simulink model "parallel_lht_accumulator"  (R2019b)
settings: Solver=FixedStepDiscrete  StartTime=0.0  StopTime=inf  RelTol=1e-3
InitFcn:
  | parallel_lht_setup;
StopFcn:
  | parallel_lht_accumulator_compare;
undefined symbols (not defined in the file or in its folder): bt, height, nTheta, width
libraries: hdlsllib x21, simulink x18, dspsrcs4 x1
(part 1 of 2)
settings Model: DataTypeOverride=Off  SimulationMode=rapid-accelerator  Creator=rgb11127  LastModifiedBy=rgb11127
settings DataIOCC: SaveOutput=off  SaveTime=off
settings OptimizationCC: BlockReduction=off  ConditionallyExecuteInputs=off  DefaultParameterBehavior=Inlined
settings DebuggingCC: AlgebraicLoopMsg=error  SingleTaskRateTransMsg=error
settings HardwareCC: ProdBitPerPointer=32  ProdBitPerSizeT=32  ProdBitPerPtrDiffT=32  ProdLargestAtomicFloat=None  ProdIntDivRoundTo=Undefined  ProdEndianess=Unspecified  ProdWordSize=32  ProdHWDeviceType=ASIC/FPGA->ASIC/FPGA  TargetBitPerPointer=64  TargetBitPerSizeT=64  TargetBitPerPtrDiffT=64  TargetLongLongMode=on  TargetIntDivRoundTo=Zero  TargetEndianess=LittleEndian  TargetWordSize=64  TargetHWDeviceType=Custom Processor->MATLAB Host Computer  ProdEqTarget=off

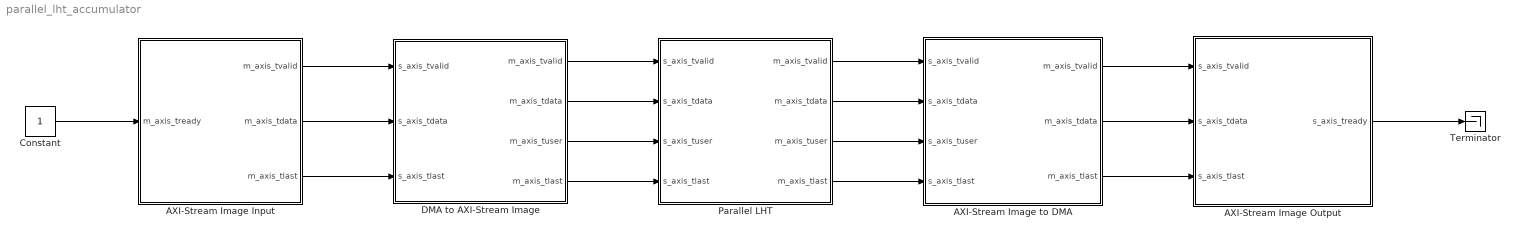
== system parallel_lht_accumulator ==
  AXI-Stream Image Input : Subsystem  mask{image=bt.inputImage, clk=1/150e6}
      mask prompts: image "Input Image:"; clk "Clock Rate:"
      mask init:
      | [height, width] = size(image);
      mask DialogControl DescGroupVar Prompt: AXI-Stream Image Input
      mask DialogControl DescTextVar Prompt: This block simulates an AXI-Stream image input for interfacing to a hardware accelerator or IP Core.
      mask DialogControl ParameterGroupVar Prompt: Main
  AXI-Stream Image Output : Subsystem  mask{height=bt.nRho, width=bt.nTheta, clk=1/150e6, d=0}
      mask prompts: height "Image Height:"; width "Image Width:"; clk "Clock Rate:"; d "Frame Capture Number"
      mask DialogControl DescGroupVar Prompt: AXI-Stream Image Output
      mask DialogControl DescTextVar Prompt: Image output using the AXI-Stream interface. Simulates an AXI DMA write channel.
      mask DialogControl ParameterGroupVar Prompt: Main
  AXI-Stream Image to DMA : Subsystem  mask{height=bt.nRho, width=bt.nTheta}
      mask prompts: height "Image Height"; width "Image Width"
      mask DialogControl DescGroupVar Prompt: AXI-Stream Image to DMA
      mask DialogControl DescTextVar Prompt: Converts from the AXI-Stream video standard to AXI-Stream DMA packet.
      mask DialogControl Container2 Prompt: Main
  Constant : Constant  OutDataTypeStr=boolean  SampleTime=-1
  DMA to AXI-Stream Image : Subsystem  mask{height=bt.height, width=bt.width, b=1}
      mask prompts: height "Image Height:"; width "Image Width:"; b "Bits"
      mask DialogControl DescGroupVar Prompt: DMA to AXI-Stream Image
      mask DialogControl DescTextVar Prompt: Converts an DMA AXI-Stream packet to the AXI-Stream video standard.
      mask DialogControl Container2 Prompt: Main
  Parallel LHT : Subsystem
  Terminator : Terminator
  wires:
  Constant/1 -> AXI-Stream Image Input/1(m_axis_tready)
  AXI-Stream Image Input/1(m_axis_tvalid) -> DMA to AXI-Stream Image/1(s_axis_tvalid)
  AXI-Stream Image Input/2(m_axis_tdata) -> DMA to AXI-Stream Image/2(s_axis_tdata)
  AXI-Stream Image Input/3(m_axis_tlast) -> DMA to AXI-Stream Image/3(s_axis_tlast)
  AXI-Stream Image to DMA/1(m_axis_tvalid) -> AXI-Stream Image Output/1(s_axis_tvalid)
  AXI-Stream Image to DMA/2(m_axis_tdata) -> AXI-Stream Image Output/2(s_axis_tdata)
  AXI-Stream Image to DMA/3(m_axis_tlast) -> AXI-Stream Image Output/3(s_axis_tlast)
  AXI-Stream Image Output/1(s_axis_tready) -> Terminator/1
  DMA to AXI-Stream Image/1(m_axis_tvalid) -> Parallel LHT/1(s_axis_tvalid)
  DMA to AXI-Stream Image/2(m_axis_tdata) -> Parallel LHT/2(s_axis_tdata)
  DMA to AXI-Stream Image/3(m_axis_tuser) -> Parallel LHT/3(s_axis_tuser)
  DMA to AXI-Stream Image/4(m_axis_tlast) -> Parallel LHT/4(s_axis_tlast)
  Parallel LHT/1(m_axis_tvalid) -> AXI-Stream Image to DMA/1(s_axis_tvalid)
  Parallel LHT/2(m_axis_tdata) -> AXI-Stream Image to DMA/2(s_axis_tdata)
  Parallel LHT/3(m_axis_tuser) -> AXI-Stream Image to DMA/3(s_axis_tuser)
  Parallel LHT/4(m_axis_tlast) -> AXI-Stream Image to DMA/4(s_axis_tlast)

== system parallel_lht_accumulator/AXI-Stream Image Input ==
  m_axis_tready : Inport
  Compare To Constant : simulink/Logic and Bit Operations/Compare To Constant  relop===  const=height*width-1  OutDataTypeStr=boolean
  Data Type Conversion : DataTypeConversion  OutDataTypeStr=uint32
  HDL Counter : hdlsllib/Sources/HDL Counter  CountType=Count limited  CountInit=0  CountStep=1  CountMax=width*height-1  CountFromType=Initial value  CountFrom=0  CountResetPort=off  CountLoadPort=off  CountEnbPort=on  CountDirPort=off  CountDataType=Unsigned  CountWordLen=ceil(log2(width*height))  CountFracLen=0  CountSampTime=1
      settings: SourceProductName=Simulink
  Master AXI-Stream FIFO : Subsystem  mask{depth=32}
      mask prompts: depth "FIFO Depth:"
      mask DialogControl DescGroupVar Prompt: Master AXI-Stream FIFO
      mask DialogControl DescTextVar Prompt: A custom AXI-Stream FIFO for interfacing to write channel AXI DMAs.
      mask DialogControl ParameterGroupVar Prompt: Main
  Synchronous Image Source : Subsystem
  m_axis_tvalid : Outport
  m_axis_tdata : Outport  Port=2
  m_axis_tlast : Outport  Port=3
  wires:
  Master AXI-Stream FIFO/2(m_axis_tdata) -> m_axis_tdata/1
  Master AXI-Stream FIFO/3(m_axis_tlast) -> m_axis_tlast/1
  m_axis_tready/1 -> Master AXI-Stream FIFO/4(m_axis_tready)
  Master AXI-Stream FIFO/4(s_axis_tready) -> HDL Counter/1, Master AXI-Stream FIFO/1(s_axis_tvalid), Synchronous Image Source/Enable
  Compare To Constant/1 -> Master AXI-Stream FIFO/3(s_axis_tlast)
  Data Type Conversion/1 -> Master AXI-Stream FIFO/2(s_axis_tdata)
  Master AXI-Stream FIFO/1(m_axis_tvalid) -> m_axis_tvalid/1
  Synchronous Image Source/1(Pixel) -> Data Type Conversion/1
  HDL Counter/1 -> Compare To Constant/1

== system parallel_lht_accumulator/AXI-Stream Image Output ==
  s_axis_tvalid : Inport
  s_axis_tdata : Inport  Port=2
  s_axis_tlast : Inport  Port=3
  AND1 : Logic  IconShape=distinctive  AllPortsSameDT=off  OutDataTypeStr=boolean
  Compare To Constant4 : simulink/Logic and Bit Operations/Compare To Constant  relop===  const=(height)*width-1  OutDataTypeStr=boolean
  Constant : Constant  OutDataTypeStr=boolean  SampleTime=-1
  Delay2 : Delay  DelayLength=d  ShowEnablePort=on
      settings: InputPortMap=u0,e6
  Pixel to Workspace : Subsystem
  Stop Simulation1 : Stop
  Terminator : Terminator
  Total Samples Counter : hdlsllib/Sources/HDL Counter  CountType=Count limited  CountInit=0  CountStep=1  CountMax=(height)*width-1  CountFromType=Initial value  CountFrom=0  CountResetPort=off  CountLoadPort=off  CountEnbPort=on  CountDirPort=off  CountDataType=Unsigned  CountWordLen=ceil(log2((height)*width+1))  CountFracLen=0  CountSampTime=1
      settings: SourceProductName=Simulink
  s_axis_tready : Outport  VectorParamsAs1DForOutWhenUnconnected=off
  wires:
  s_axis_tdata/1 -> Pixel to Workspace/1(Pixel In)
  s_axis_tvalid/1 -> AND1/1
  AND1/1 -> Total Samples Counter/1, Pixel to Workspace/Enable
  Total Samples Counter/1 -> Compare To Constant4/1
  Compare To Constant4/1 -> Delay2/2, Delay2/1
  Delay2/1 -> Stop Simulation1/1
  s_axis_tlast/1 -> Terminator/1
  Constant/1 -> AND1/2, s_axis_tready/1

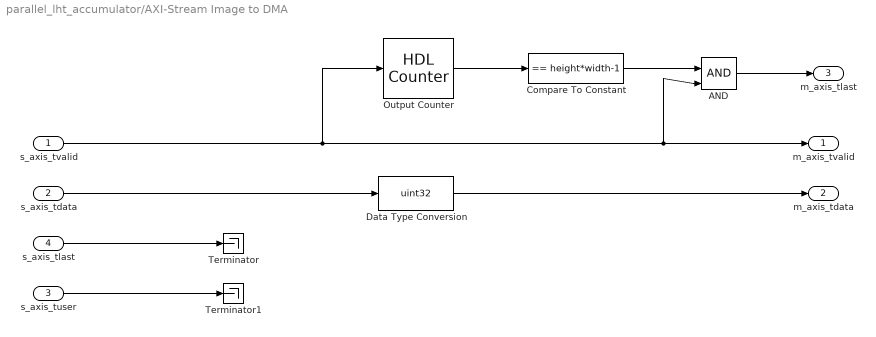
== system parallel_lht_accumulator/AXI-Stream Image to DMA ==
  s_axis_tvalid : Inport
  s_axis_tdata : Inport  Port=2
  s_axis_tuser : Inport  Port=3
  s_axis_tlast : Inport  Port=4
  AND : Logic  IconShape=distinctive  AllPortsSameDT=off  OutDataTypeStr=boolean
  Compare To Constant : simulink/Logic and Bit Operations/Compare To Constant  relop===  const=height*width-1  OutDataTypeStr=boolean
  Data Type Conversion : DataTypeConversion  OutDataTypeStr=uint32
  Output Counter : hdlsllib/Sources/HDL Counter  CountType=Count limited  CountInit=0  CountStep=1  CountMax=height*width-1  CountFromType=Initial value  CountFrom=0  CountResetPort=off  CountLoadPort=off  CountEnbPort=on  CountDirPort=off  CountDataType=Unsigned  CountWordLen=ceil(log2(height*width))  CountFracLen=0  CountSampTime=1
      settings: SourceProductName=Simulink
  Terminator : Terminator
  Terminator1 : Terminator
  m_axis_tvalid : Outport
  m_axis_tdata : Outport  Port=2
  m_axis_tlast : Outport  Port=3
  wires:
  AND/1 -> m_axis_tlast/1
  Compare To Constant/1 -> AND/1
  Output Counter/1 -> Compare To Constant/1
  s_axis_tuser/1 -> Terminator1/1
  s_axis_tlast/1 -> Terminator/1
  s_axis_tvalid/1 -> Output Counter/1, m_axis_tvalid/1, AND/2
  s_axis_tdata/1 -> Data Type Conversion/1
  Data Type Conversion/1 -> m_axis_tdata/1

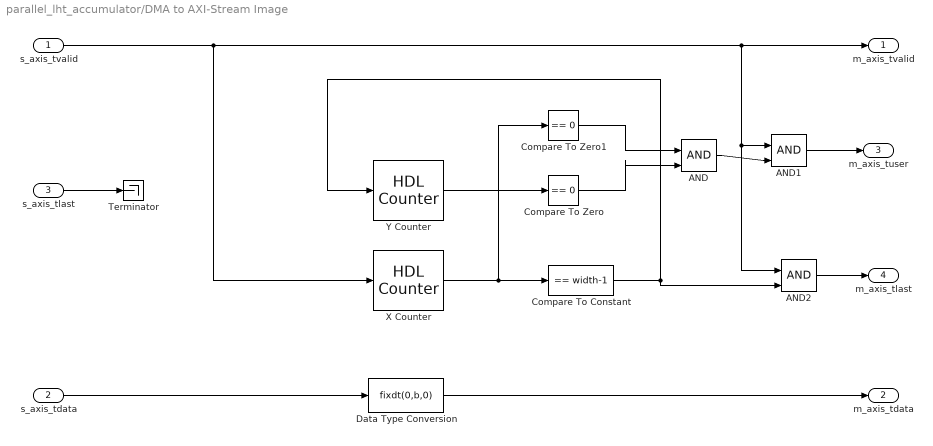
== system parallel_lht_accumulator/DMA to AXI-Stream Image ==
  s_axis_tvalid : Inport
  s_axis_tdata : Inport  Port=2
  s_axis_tlast : Inport  Port=3
  AND : Logic  IconShape=distinctive  AllPortsSameDT=off  OutDataTypeStr=boolean
  AND1 : Logic  IconShape=distinctive  AllPortsSameDT=off  OutDataTypeStr=boolean
  AND2 : Logic  IconShape=distinctive  AllPortsSameDT=off  OutDataTypeStr=boolean
  Compare To Constant : simulink/Logic and Bit Operations/Compare To Constant  relop===  const=width-1  OutDataTypeStr=boolean
  Compare To Zero : simulink/Logic and Bit Operations/Compare To Zero  relop===  OutDataTypeStr=boolean
  Compare To Zero1 : simulink/Logic and Bit Operations/Compare To Zero  relop===  OutDataTypeStr=boolean
  Data Type Conversion : DataTypeConversion  OutDataTypeStr=fixdt(0,b,0)  ConvertRealWorld=Stored Integer (SI)
  Terminator : Terminator
  X Counter : hdlsllib/Sources/HDL Counter  CountType=Count limited  CountInit=0  CountStep=1  CountMax=width-1  CountFromType=Initial value  CountFrom=0  CountResetPort=off  CountLoadPort=off  CountEnbPort=on  CountDirPort=off  CountDataType=Unsigned  CountWordLen=ceil(log2(width))  CountFracLen=0  CountSampTime=1
      settings: SourceProductName=Simulink
  Y Counter : hdlsllib/Sources/HDL Counter  CountType=Count limited  CountInit=0  CountStep=1  CountMax=height-1  CountFromType=Initial value  CountFrom=0  CountResetPort=off  CountLoadPort=off  CountEnbPort=on  CountDirPort=off  CountDataType=Unsigned  CountWordLen=ceil(log2(height))  CountFracLen=0  CountSampTime=1
      settings: SourceProductName=Simulink
  m_axis_tvalid : Outport
  m_axis_tdata : Outport  Port=2
  m_axis_tuser : Outport  Port=3
  m_axis_tlast : Outport  Port=4
  wires:
  AND2/1 -> m_axis_tlast/1
  Compare To Constant/1 -> Y Counter/1, AND2/2
  AND1/1 -> m_axis_tuser/1
  AND/1 -> AND1/2
  s_axis_tdata/1 -> Data Type Conversion/1
  Compare To Zero/1 -> AND/2
  Compare To Zero1/1 -> AND/1
  Y Counter/1 -> Compare To Zero/1
  X Counter/1 -> Compare To Constant/1, Compare To Zero1/1
  s_axis_tvalid/1 -> m_axis_tvalid/1, AND1/1, AND2/1, X Counter/1
  Data Type Conversion/1 -> m_axis_tdata/1
  s_axis_tlast/1 -> Terminator/1

== system parallel_lht_accumulator/Parallel LHT ==
  s_axis_tvalid : Inport
  s_axis_tdata : Inport  Port=2
  s_axis_tuser : Inport  Port=3
  s_axis_tlast : Inport  Port=4
  Parallel LHT Accumulator : Subsystem  mask{height=bt.height, width=bt.width, theta=bt.theta}
      mask prompts: height "Image Height:"; width "Image Width:"; theta "Orientations:"
      mask init:
      | maxRho = ceil(sqrt((height/2)^2+(width/2)^2));
      | nRho = maxRho*2;
      | [~, nTheta] = size(theta);
      mask DialogControl ParameterGroupVar Prompt: Main
  Parallel LHT Kernel : Subsystem  mask{height=bt.height, width=bt.width, theta=bt.theta, kFlag=Symmetric Look Ahead}
      mask prompts: height "Image Height:"; width "Image Width:"; theta "Orientations:"; kFlag "Kernel Architecture:"
      mask init:
      | maxRho = ceil(sqrt((height/2)^2+(width/2)^2));
      | [~, nTheta] = size(theta);
      | nRho = maxRho*2;
      | 
      | blk = [gcb '/Hough Kernel'];
      | 
      | oldVariant = get_param(blk,'OverrideUsingVariant');
      | 
      | switch get_param(gcb, 'kFlag')
      |     case 'Parallel'
      |         newVariant = 'Parallel';
      |     case 'Symmetric'
      |         newVariant = 'Symmetric';
      |     case 'Symmetric Look Ahead'
      |         newVariant = 'SymmetricLookAhead';
      |     otherwise
      |         newVariant = 'Simple';
      | end
      | 
      | if ~strcmp(oldVariant, newVariant)
      |     set_param(blk, 'OverrideUsingVariant', newVariant);
      | end
      mask TypeOptions kFlag: Parallel | Symmetric | Symmetric Look Ahead
      mask DialogControl ParameterGroupVar Prompt: Main
  m_axis_tvalid : Outport
  m_axis_tdata : Outport  Port=2
  m_axis_tuser : Outport  Port=3
  m_axis_tlast : Outport  Port=4
  wires:
  Parallel LHT Kernel/4(m_axis_tlast) -> Parallel LHT Accumulator/4(s_axis_tlast)
  Parallel LHT Accumulator/4(m_axis_tlast) -> m_axis_tlast/1
  Parallel LHT Accumulator/1(m_axis_tvalid) -> m_axis_tvalid/1
  Parallel LHT Kernel/5(hough_param) -> Parallel LHT Accumulator/5(hough_param)
  Parallel LHT Kernel/2(m_axis_tdata) -> Parallel LHT Accumulator/2(s_axis_tdata)
  s_axis_tlast/1 -> Parallel LHT Kernel/4(s_axis_tlast)
  Parallel LHT Kernel/1(m_axis_tvalid) -> Parallel LHT Accumulator/1(s_axis_tvalid)
  s_axis_tdata/1 -> Parallel LHT Kernel/2(s_axis_tdata)
  Parallel LHT Kernel/3(m_axis_tuser) -> Parallel LHT Accumulator/3(s_axis_tuser)
  Parallel LHT Accumulator/3(m_axis_tuser) -> m_axis_tuser/1
  Parallel LHT Accumulator/2(m_axis_tdata) -> m_axis_tdata/1
  s_axis_tuser/1 -> Parallel LHT Kernel/3(s_axis_tuser)
  s_axis_tvalid/1 -> Parallel LHT Kernel/1(s_axis_tvalid)

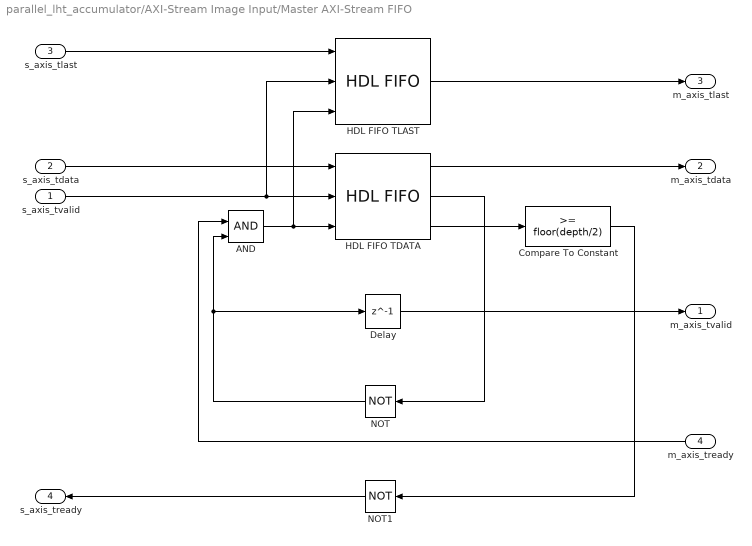
== system parallel_lht_accumulator/AXI-Stream Image Input/Master AXI-Stream FIFO ==
  s_axis_tvalid : Inport
  s_axis_tdata : Inport  Port=2
  s_axis_tlast : Inport  Port=3
  m_axis_tready : Inport  Port=4
  AND : Logic  IconShape=distinctive  AllPortsSameDT=off  OutDataTypeStr=boolean
  "Compare To Constant " : simulink/Logic and Bit Operations/Compare To Constant  relop=>=  const=floor(depth/2)  OutDataTypeStr=boolean
  Delay : Delay  DelayLength=1
  HDL FIFO TDATA : hdlsllib/HDL RAMs/HDL FIFO  fifo_size=depth  mode=Classic  ratio=1  push_msg=Error  pop_msg=Error  show_empty=on  show_full=off  show_num=on  LabelModeActiveChoice_Mode=Classic
      settings: SourceProductName=Simulink  SourceProductBaseCode=SL
  HDL FIFO TLAST : hdlsllib/HDL RAMs/HDL FIFO  fifo_size=depth  mode=Classic  ratio=1  push_msg=Error  pop_msg=Error  show_empty=off  show_full=off  show_num=off  LabelModeActiveChoice_Mode=Classic
      settings: SourceProductName=Simulink  SourceProductBaseCode=SL
  NOT : Logic  Operator=NOT  IconShape=distinctive  AllPortsSameDT=off  OutDataTypeStr=boolean
  NOT1 : Logic  Operator=NOT  IconShape=distinctive  AllPortsSameDT=off  OutDataTypeStr=boolean
  m_axis_tvalid : Outport  VectorParamsAs1DForOutWhenUnconnected=off
  m_axis_tdata : Outport  Port=2  VectorParamsAs1DForOutWhenUnconnected=off
  m_axis_tlast : Outport  Port=3  VectorParamsAs1DForOutWhenUnconnected=off
  s_axis_tready : Outport  Port=4
  wires:
  Delay/1 -> m_axis_tvalid/1
  s_axis_tvalid/1 -> HDL FIFO TDATA/2, HDL FIFO TLAST/2
  s_axis_tdata/1 -> HDL FIFO TDATA/1
  s_axis_tlast/1 -> HDL FIFO TLAST/1
  "Compare To Constant "/1 -> NOT1/1
  NOT1/1 -> s_axis_tready/1
  HDL FIFO TDATA/3 -> "Compare To Constant "/1
  m_axis_tready/1 -> AND/1
  NOT/1 -> AND/2, Delay/1
  AND/1 -> HDL FIFO TDATA/3, HDL FIFO TLAST/3
  HDL FIFO TDATA/2 -> NOT/1
  HDL FIFO TLAST/1 -> m_axis_tlast/1
  HDL FIFO TDATA/1 -> m_axis_tdata/1

== system parallel_lht_accumulator/AXI-Stream Image Input/Synchronous Image Source ==
  Enable : EnablePort
  Signal From Workspace : dspsrcs4/Signal From Workspace  X=reshape(image', [height*width, 1])  Ts=clk  nsamps=1  OutputAfterFinalValue=Cyclic repetition  ignoreOrWarnInputAndFrameLengths=off  OutputFrames=off
  Pixel : Outport
  wires:
  Signal From Workspace/1 -> Pixel/1

== system parallel_lht_accumulator/AXI-Stream Image Output/Pixel to Workspace ==
  Pixel In : Inport
  Enable : EnablePort
  To Workspace : ToWorkspace  VariableName=simout  SampleTime=-1
      settings: MaxDataPoints=height*width  Save2DSignal=2-D array (concatenate along first dimension)
  wires:
  Pixel In/1 -> To Workspace/1

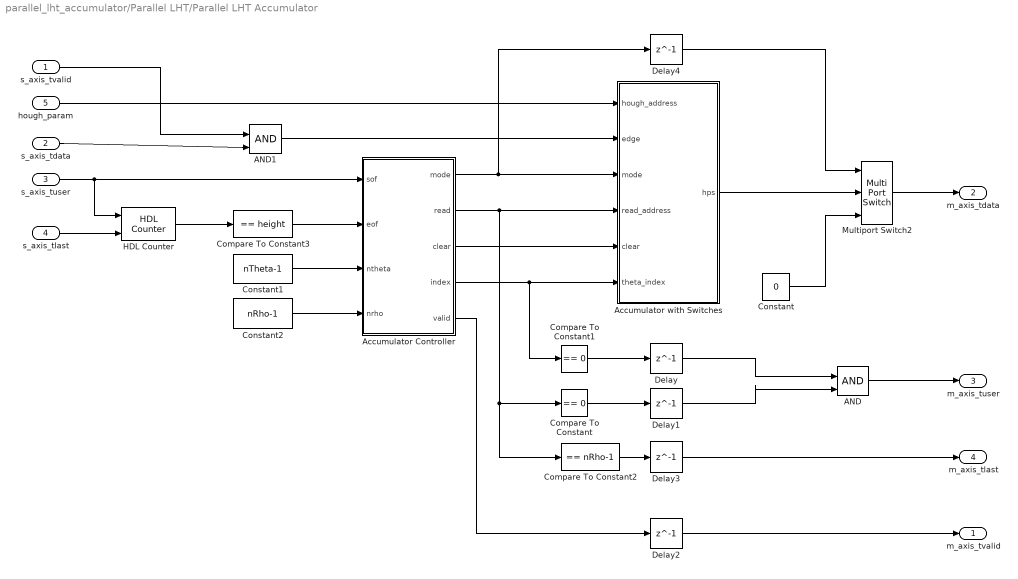
== system parallel_lht_accumulator/Parallel LHT/Parallel LHT Accumulator ==
  s_axis_tvalid : Inport
  s_axis_tdata : Inport  Port=2
  s_axis_tuser : Inport  Port=3
  s_axis_tlast : Inport  Port=4
  hough_param : Inport  Port=5
  AND : Logic  IconShape=distinctive  AllPortsSameDT=off  OutDataTypeStr=boolean
  AND1 : Logic  IconShape=distinctive  AllPortsSameDT=off  OutDataTypeStr=boolean
  Accumulator Controller : MATLAB Function  TreatAsAtomicUnit=on
  Accumulator with Switches : Subsystem
  Compare To Constant : simulink/Logic and Bit Operations/Compare To Constant  relop===  const=0  OutDataTypeStr=boolean
  Compare To Constant1 : simulink/Logic and Bit Operations/Compare To Constant  relop===  const=0  OutDataTypeStr=boolean
  Compare To Constant2 : simulink/Logic and Bit Operations/Compare To Constant  relop===  const=nRho-1  OutDataTypeStr=boolean
  Compare To Constant3 : simulink/Logic and Bit Operations/Compare To Constant  relop===  const=height  OutDataTypeStr=boolean
  Constant : Constant  Value=0  OutDataTypeStr=fixdt(0, ceil(log2(2*maxRho)), 0)  SampleTime=-1
  Constant1 : Constant  Value=nTheta-1  OutDataTypeStr=uint16  SampleTime=-1
  Constant2 : Constant  Value=nRho-1  OutDataTypeStr=uint16  SampleTime=-1
  Delay{,1..4} (5 alike) : Delay  DelayLength=1
  HDL Counter : hdlsllib/Sources/HDL Counter  CountType=Count limited  CountInit=0  CountStep=1  CountMax=height  CountFromType=Initial value  CountFrom=0  CountResetPort=on  CountLoadPort=off  CountEnbPort=on  CountDirPort=off  CountDataType=Unsigned  CountWordLen=ceil(log2(height+1))  CountFracLen=0  CountSampTime=1
      settings: SourceProductName=Simulink
  Multiport Switch2 : MultiPortSwitch  DataPortOrder=Zero-based contiguous  Inputs=2  zeroidx=on
  m_axis_tvalid : Outport
  m_axis_tdata : Outport  Port=2
  m_axis_tuser : Outport  Port=3
  m_axis_tlast : Outport  Port=4
  wires:
  Accumulator Controller/3(clear) -> Accumulator with Switches/5(clear)
  Accumulator Controller/1(mode) -> Delay4/1, Accumulator with Switches/3(mode)
  Accumulator Controller/2(read) -> Compare To Constant2/1, Compare To Constant/1, Accumulator with Switches/4(read_address)
  Constant1/1 -> Accumulator Controller/3(ntheta)
  Accumulator Controller/4(index) -> Compare To Constant1/1, Accumulator with Switches/6(theta_index)
  Compare To Constant2/1 -> Delay3/1
  Constant2/1 -> Accumulator Controller/4(nrho)
  s_axis_tuser/1 -> HDL Counter/1, Accumulator Controller/1(sof)
  Delay/1 -> AND/1
  Delay1/1 -> AND/2
  Compare To Constant1/1 -> Delay/1
  Compare To Constant/1 -> Delay1/1
  Delay3/1 -> m_axis_tlast/1
  hough_param/1 -> Accumulator with Switches/1(hough_address)
  AND/1 -> m_axis_tuser/1
  s_axis_tdata/1 -> AND1/2
  AND1/1 -> Accumulator with Switches/2(edge)
  s_axis_tvalid/1 -> AND1/1
  HDL Counter/1 -> Compare To Constant3/1
  s_axis_tlast/1 -> HDL Counter/2
  Compare To Constant3/1 -> Accumulator Controller/2(eof)
  Multiport Switch2/1 -> m_axis_tdata/1
  Accumulator with Switches/1(hps) -> Multiport Switch2/2
  Constant/1 -> Multiport Switch2/3
  Accumulator Controller/5(valid) -> Delay2/1
  Delay2/1 -> m_axis_tvalid/1
  Delay4/1 -> Multiport Switch2/1

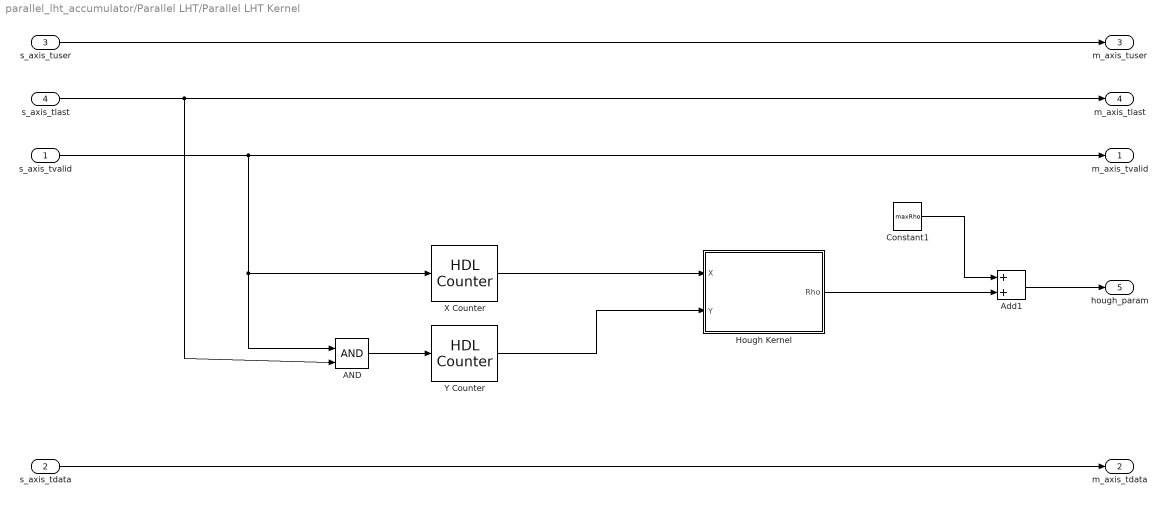
== system parallel_lht_accumulator/Parallel LHT/Parallel LHT Kernel ==
  s_axis_tvalid : Inport
  s_axis_tdata : Inport  Port=2
  s_axis_tuser : Inport  Port=3
  s_axis_tlast : Inport  Port=4
  AND : Logic  IconShape=distinctive  AllPortsSameDT=off  OutDataTypeStr=boolean
  Add1 : Sum  OutDataTypeStr=fixdt(0, ceil(log2(2*maxRho+1)), 0);  RndMeth=Round
  Constant1 : Constant  Value=maxRho  OutDataTypeStr=fixdt(0, ceil(log2(maxRho + 1)), 0);  SampleTime=-1
  Hough Kernel : Subsystem  VariantControlMode=Label  Variant=on  VariantControl=Variant1  LabelModeActiveChoice=SymmetricLookAhead
  X Counter : hdlsllib/Sources/HDL Counter  CountType=Count limited  CountInit=-width/2  CountStep=1  CountMax=width/2-1  CountFromType=Initial value  CountFrom=-width/2  CountResetPort=off  CountLoadPort=off  CountEnbPort=on  CountDirPort=off  CountDataType=Signed  CountWordLen=ceil(log2(width))  CountFracLen=0  CountSampTime=1
      settings: SourceProductName=Simulink
  Y Counter : hdlsllib/Sources/HDL Counter  CountType=Count limited  CountInit=-height/2  CountStep=1  CountMax=height/2-1  CountFromType=Initial value  CountFrom=-height/2  CountResetPort=off  CountLoadPort=off  CountEnbPort=on  CountDirPort=off  CountDataType=Signed  CountWordLen=ceil(log2(height))  CountFracLen=0  CountSampTime=1
      settings: SourceProductName=Simulink
  m_axis_tvalid : Outport
  m_axis_tdata : Outport  Port=2
  m_axis_tuser : Outport  Port=3
  m_axis_tlast : Outport  Port=4
  hough_param : Outport  Port=5
  wires:
  s_axis_tvalid/1 -> X Counter/1, AND/1, m_axis_tvalid/1
  AND/1 -> Y Counter/1
  s_axis_tlast/1 -> AND/2, m_axis_tlast/1
  s_axis_tdata/1 -> m_axis_tdata/1
  s_axis_tuser/1 -> m_axis_tuser/1
  Add1/1 -> hough_param/1
  Constant1/1 -> Add1/1
  X Counter/1 -> Hough Kernel/1(X)
  Y Counter/1 -> Hough Kernel/2(Y)
  Hough Kernel/1(Rho) -> Add1/2

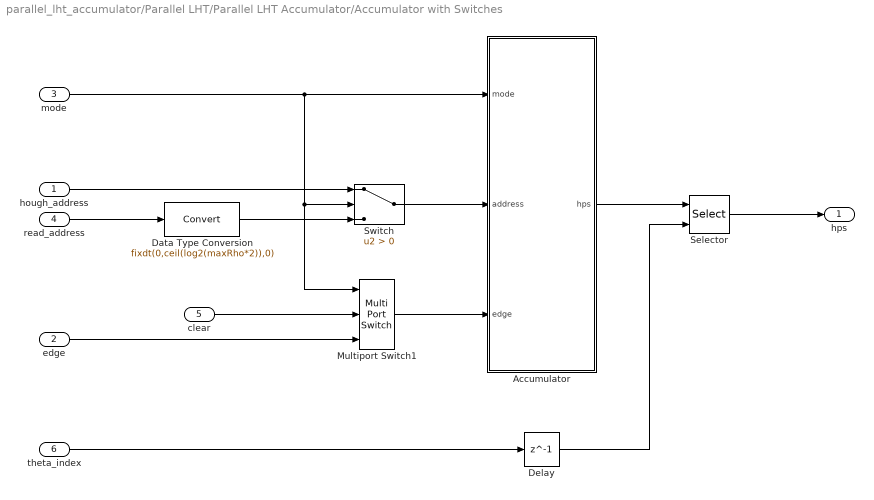
== system parallel_lht_accumulator/Parallel LHT/Parallel LHT Accumulator/Accumulator with Switches ==
  hough_address : Inport
  edge : Inport  Port=2
  mode : Inport  Port=3
  read_address : Inport  Port=4
  clear : Inport  Port=5
  theta_index : Inport  Port=6
  Accumulator : Subsystem
  Data Type Conversion : DataTypeConversion  OutDataTypeStr=fixdt(0,ceil(log2(maxRho*2)),0)
  Delay : Delay  DelayLength=1
  Multiport Switch1 : MultiPortSwitch  DataPortOrder=Zero-based contiguous  Inputs=2  zeroidx=on
  Selector : Selector  NumberOfDimensions=2  IndexMode=Zero-based  InputPortWidth=3  IndexOptions=Index vector (dialog),Index vector (port)  Indices=0,0  OutputSizes=1,1
  Switch : Switch  Criteria=u2 > Threshold
  hps : Outport
  wires:
  Accumulator/1(hps) -> Selector/1
  mode/1 -> Switch/2, Multiport Switch1/1, Accumulator/1(mode)
  read_address/1 -> Data Type Conversion/1
  Switch/1 -> Accumulator/2(address)
  Multiport Switch1/1 -> Accumulator/3(edge)
  hough_address/1 -> Switch/1
  theta_index/1 -> Delay/1
  Selector/1 -> hps/1
  edge/1 -> Multiport Switch1/3
  clear/1 -> Multiport Switch1/2
  Data Type Conversion/1 -> Switch/3
  Delay/1 -> Selector/2

== system parallel_lht_accumulator/Parallel LHT/Parallel LHT Kernel/Hough Kernel ==
  X : Inport
  Y : Inport  Port=2
  Hough Kernel Parallel : Subsystem  VariantControl=Parallel
  Hough Kernel Symmetric : Subsystem  VariantControl=Symmetric
  Hough Kernel Symmetric Look Ahead : Subsystem  VariantControl=SymmetricLookAhead
  Rho : Outport

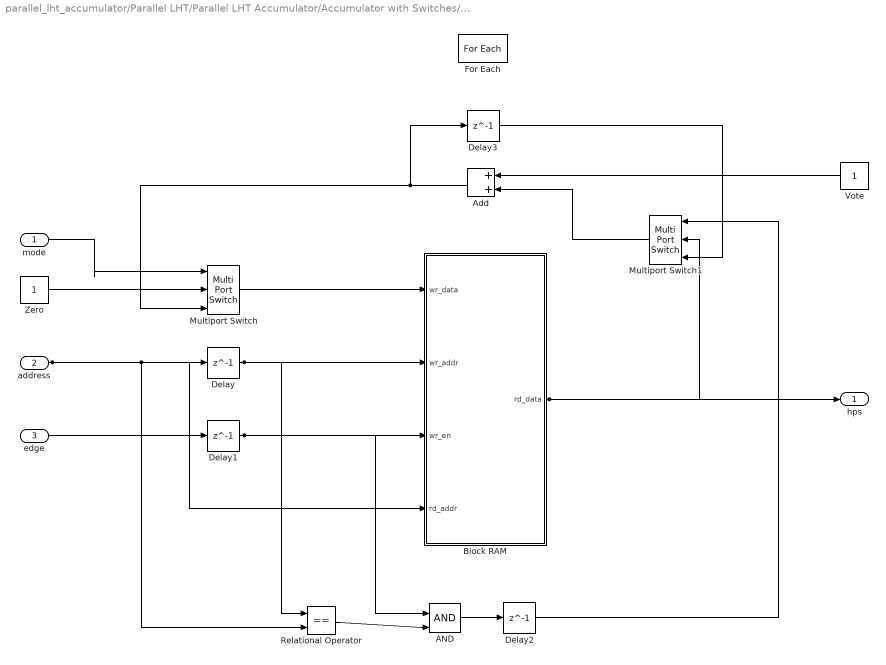
== system parallel_lht_accumulator/Parallel LHT/Parallel LHT Accumulator/Accumulator with Switches/Accumulator ==
  mode : Inport
  address : Inport  Port=2  Partition=on  PartitionDimension=2  PartitionWidth=1  PartitionOffset=0
  edge : Inport  Port=3
  AND : Logic  IconShape=distinctive  AllPortsSameDT=off  OutDataTypeStr=boolean
  Add : Sum  OutDataTypeStr=fixdt(0, ceil(log2(maxRho*2)), 0)
  Block RAM : Subsystem  VariantControlMode=Label  Variant=on  VariantControl=Variant1  LabelModeActiveChoice=other_bits
  Delay{,1..3} (4 alike) : Delay  DelayLength=1
  For Each : ForEach  DisableCoverage=on
  Multiport Switch : MultiPortSwitch  DataPortOrder=Zero-based contiguous  Inputs=2  zeroidx=on
  Multiport Switch1 : MultiPortSwitch  DataPortOrder=Zero-based contiguous  Inputs=2  zeroidx=on
  Relational Operator : RelationalOperator  Operator===  OutDataTypeStr=boolean  RndMeth=Simplest
  Vote : Constant  OutDataTypeStr=fixdt(0,1,0)  SampleTime=-1
  Zero : Constant  OutDataTypeStr=fixdt(0,1,0)  SampleTime=-1
  hps : Outport  ConcatenationDimension=2
  wires:
  Relational Operator/1 -> AND/2
  Delay/1 -> Relational Operator/1, Block RAM/2(wr_addr)
  Delay2/1 -> Multiport Switch1/1
  address/1 -> Delay/1, Relational Operator/2, Block RAM/4(rd_addr)
  AND/1 -> Delay2/1
  Delay1/1 -> AND/1, Block RAM/3(wr_en)
  Add/1 -> Multiport Switch/3, Delay3/1
  Multiport Switch1/1 -> Add/2
  Vote/1 -> Add/1
  Delay3/1 -> Multiport Switch1/3
  Zero/1 -> Multiport Switch/2
  edge/1 -> Delay1/1
  mode/1 -> Multiport Switch/1
  Multiport Switch/1 -> Block RAM/1(wr_data)
  Block RAM/1(rd_data) -> Multiport Switch1/2, hps/1

== system parallel_lht_accumulator/Parallel LHT/Parallel LHT Kernel/Hough Kernel/Hough Kernel Parallel ==
  X : Inport
  Y : Inport  Port=2
  Add : Sum  OutDataTypeStr=fixdt(1,ceil(log2(maxRho*2+1)),0)  RndMeth=Round
  Cosine : Constant  Value=fi(cos(deg2rad(theta)), 1, 16, 14)  VectorParams1D=off  OutDataTypeStr=fixdt(1,16,14)  SampleTime=-1
  Sine : Constant  Value=fi(sin(deg2rad(theta)), 1, 16, 14)  VectorParams1D=off  OutDataTypeStr=fixdt(1,16,14)  SampleTime=-1
  xcos : Product  OutDataTypeStr=fixdt(1, ceil(log2(width)), 0)  RndMeth=Round
  ysin : Product  OutDataTypeStr=fixdt(1, ceil(log2(height)), 0)  RndMeth=Round
  Rho : Outport
  wires:
  Cosine/1 -> xcos/1
  Y/1 -> ysin/1
  ysin/1 -> Add/2
  X/1 -> xcos/2
  xcos/1 -> Add/1
  Sine/1 -> ysin/2
  Add/1 -> Rho/1

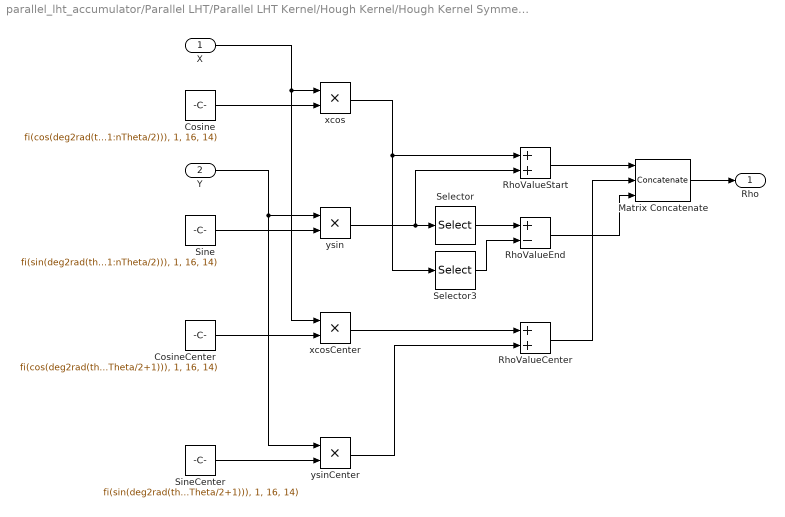
== system parallel_lht_accumulator/Parallel LHT/Parallel LHT Kernel/Hough Kernel/Hough Kernel Symmetric ==
  X : Inport
  Y : Inport  Port=2
  Cosine : Constant  Value=fi(cos(deg2rad(theta(1:nTheta/2))), 1, 16, 14)  VectorParams1D=off  OutDataTypeStr=fixdt(1,16,14)  SampleTime=-1
  CosineCenter : Constant  Value=fi(cos(deg2rad(theta(nTheta/2+1))), 1, 16, 14)  VectorParams1D=off  OutDataTypeStr=fixdt(1,16,14)  SampleTime=-1
  Matrix Concatenate : Concatenate  NumInputs=3  Mode=Multidimensional array  ConcatenateDimension=2
  RhoValueCenter : Sum  OutDataTypeStr=fixdt(1, ceil(log2(2*maxRho)), 0);  RndMeth=Round
  RhoValueEnd : Sum  Inputs=+-  OutDataTypeStr=fixdt(1, ceil(log2(2*maxRho)), 0);  RndMeth=Round
  RhoValueStart : Sum  OutDataTypeStr=fixdt(1, ceil(log2(2*maxRho)), 0);  RndMeth=Round
  Selector : Selector  NumberOfDimensions=2  IndexMode=Zero-based  InputPortWidth=3  IndexOptions=Index vector (dialog),Index vector (dialog)  Indices=0,uint32([nTheta/2-1:-1:1])  OutputSizes=1,1
  Selector3 : Selector  NumberOfDimensions=2  IndexMode=Zero-based  InputPortWidth=3  IndexOptions=Index vector (dialog),Index vector (dialog)  Indices=0,uint32([nTheta/2-1:-1:1])  OutputSizes=1,1
  Sine : Constant  Value=fi(sin(deg2rad(theta(1:nTheta/2))), 1, 16, 14)  VectorParams1D=off  OutDataTypeStr=fixdt(1,16,14)  SampleTime=-1
  SineCenter : Constant  Value=fi(sin(deg2rad(theta(nTheta/2+1))), 1, 16, 14)  VectorParams1D=off  OutDataTypeStr=fixdt(1,16,14)  SampleTime=-1
  xcos : Product  OutDataTypeStr=fixdt(1, ceil(log2(width)), 0);  RndMeth=Round
  xcosCenter : Product  OutDataTypeStr=fixdt(1, ceil(log2(width)), 0);  RndMeth=Round
  ysin : Product  OutDataTypeStr=fixdt(1, ceil(log2(height)), 0);  RndMeth=Round
  ysinCenter : Product  OutDataTypeStr=fixdt(1, ceil(log2(height)), 0);  RndMeth=Round
  Rho : Outport  VectorParamsAs1DForOutWhenUnconnected=off
  wires:
  Selector3/1 -> RhoValueEnd/2
  Selector/1 -> RhoValueEnd/1
  xcos/1 -> RhoValueStart/1, Selector3/1
  Y/1 -> ysinCenter/1, ysin/1
  ysin/1 -> RhoValueStart/2, Selector/1
  Sine/1 -> ysin/2
  Cosine/1 -> xcos/2
  CosineCenter/1 -> xcosCenter/2
  SineCenter/1 -> ysinCenter/2
  X/1 -> xcosCenter/1, xcos/1
  xcosCenter/1 -> RhoValueCenter/1
  ysinCenter/1 -> RhoValueCenter/2
  Matrix Concatenate/1 -> Rho/1
  RhoValueStart/1 -> Matrix Concatenate/1
  RhoValueCenter/1 -> Matrix Concatenate/2
  RhoValueEnd/1 -> Matrix Concatenate/3

== system parallel_lht_accumulator/Parallel LHT/Parallel LHT Kernel/Hough Kernel/Hough Kernel Symmetric Look Ahead ==
  X : Inport
  Y : Inport  Port=2
  Compare To Constant1 : simulink/Logic and Bit Operations/Compare To Constant  relop===  const=width/2-1  OutDataTypeStr=boolean
  Hough Kernel Symmetric : Subsystem
  Look Ahead Hough : Subsystem
  Rho : Outport  VectorParamsAs1DForOutWhenUnconnected=off
  wires:
  X/1 -> Compare To Constant1/1, Hough Kernel Symmetric/1(X)
  Hough Kernel Symmetric/1(Rho) -> Rho/1
  Compare To Constant1/1 -> Look Ahead Hough/2(eol)
  Look Ahead Hough/1(ysin) -> Hough Kernel Symmetric/2(ysin)
  Y/1 -> Look Ahead Hough/1(Y)

== system parallel_lht_accumulator/Parallel LHT/Parallel LHT Accumulator/Accumulator with Switches/Accumulator/Block RAM ==
  wr_data : Inport
  wr_addr : Inport  Port=2
  wr_en : Inport  Port=3
  rd_addr : Inport  Port=4
  Simple Dual Port RAM : Subsystem  VariantControl=9_bits
  Simple Dual Port RAM Generator : Subsystem  VariantControl=other_bits  mask{b=12, d=2204, b_hidden=12, d_hidden=2204}
      mask prompts: b "Data width:"; d "Depth:"
      mask init:
      | if b == b_hidden && d == d_hidden
      |     return
      | end
      | 
      | % Xilinx RAM Initialisation
      | xl_config = [512, 72;
      |             1024, 36;
      |             2048, 18;
      |             4096, 9;
      |             8192, 4;
      |             16384, 2;
      |             32768, 1];
      | 
      | % Get length of Xilinx Configuration
      | sizeram = size(xl_config);
      |         
      | % Get the RAM Configuration based on the data width
      | for i = 1:sizeram(1)
      |     if b <= xl_config(i, 2)
      |         a = xl_config(i, :);
      |     end
      | end
      | 
      | % Get number of BRAM required (including half BRAM)
      | numbram = ceil((d/a(1))/0.5)*0.5;
      | fullbram = floor(numbram); % Integer
      | halfbram = (numbram-floor(numbram)) ~= 0; % Boolean
      | 
      | % Get all blocks and delete everything excepts ports
      | H = get(find_system(gcb, 'FindAll', 'on', 'type', 'block'));
      | todelete = setdiff(strcat(repmat({[gcb '/']}, numel(H.Blocks), 1),  H.Blocks),...
      |     strcat(repmat({[gcb '/']}, 5, 1),...
      |     {'wr_data'; 'wr_addr'; 'wr_en'; 'rd_addr'; 'rd_data'}));
      | delete_block(todelete);
      | 
      | % Delete lines
      | for i = 1:numel(H.Lines)
      |     delete_line(H.Lines(i).Handle)
      | end
      | 
      | % Generate full BRAMs
      | y = 0;
      | 
      | % If there is only one ram then the write enable should be directly
      | % connected to the first ram write enable. Else, the write address must be sliced
      | % and the upper bound (over a(2)) compared to zero. This will indicate if
      | % the first ram is the one to be written/read from.
      | 
      | % Common to both implementations
      | % Write Address Slice
      | add_block('hdlsllib/Logic and Bit Operations/Bit Slice',...
      |         [gcb, '/wr_address'], 'Position',...
      |         [160 130 250 170]);
      | % Set bitslice parameters
      | set_param([gcb, '/wr_address'],...
      |     'lidx', int2str(log2(a(1))-1));
      | set_param([gcb, '/wr_address'],...
      |     'ridx', int2str(0));
      | 
      | % Read Address Slice
      | add_block('hdlsllib/Logic and Bit Operations/Bit Slice',...
      |         [gcb, '/rd_address'], 'Position',...
      |         [160 330 250 370]);
      | % Set bitslice parameters
      | set_param([gcb, '/rd_address'],...
      |     'lidx', int2str(log2(a(1))-1));
      | set_param([gcb, '/rd_address'],...
      |     'ridx', int2str(0));
      | 
      | if ceil(numbram) == 1
      |     
      |     i = 1;
      |     
      |     % Add Simple RAM
      |     add_block('hdlsllib/HDL RAMs/Simple Dual Port RAM',...
      |         [gcb, '/simple_ram_', int2str(i-1)], 'Position',...
      |         [635 0+600*y 635+200 400+600*y]);
      | 
      |     % Set RAM parameters
      |     set_param([gcb, '/simple_ram_', int2str(i-1)],...
      |         'ram_size', int2str(log2(a(1))));
      | 
      |     % Connect "wr_data" to "simple_ram_i"
      |     add_line(gcb, ['wr_data/1'], ['simple_ram_', int2str(i-1), '/1'],...
      |         'autorouting', 'on');
      |     
      |     % Connect "wr_addr" to "wr_address"
      |     add_line(gcb, ['wr_addr/1'], ['wr_address/1'],...
      |         'autorouting', 'on');
      | 
      |     % Connect "wr_address" to "simple_ram_i"
      |     add_line(gcb, ['wr_address/1'], ['simple_ram_', int2str(i-1), '/2'],...
      |         'autorouting', 'on');
      | 
      |     % Connect "wr_en" to "simple_ram_i"
      |     add_line(gcb, ['wr_en/1'], ['simple_ram_', int2str(i-1), '/3'],...
      |         'autorouting', 'on');
      |     
      |     % Connect "rd_addr" to "rd_address"
      |     add_line(gcb, ['rd_addr/1'], ['rd_address/1'],...
      |         'autorouting', 'on');
      | 
      |     % Connect "rd_address" to "simple_ram_i"
      |     add_line(gcb, ['rd_address/1'], ['simple_ram_', int2str(i-1), '/4'],...
      |         'autorouting', 'on');
      | 
      |     % Connect "simple_ram_i" to "rd_data"
      |     add_line(gcb, ['simple_ram_', int2str(i-1), '/1'], ['rd_data/1'],...
      |         'autorouting', 'on');
      | 
      | else
      |     
      |     % Multiport Switch
      |     add_block('hdlsllib/Signal Routing/Multiport Switch',...
      |         [gcb, '/multiport_switch'], 'Position',...
      |         [1340 146 1405 250]);
      |     % Set multiport switch parameters
      |     set_param([gcb, '/multiport_switch'],...
      |         'Inputs', int2str(ceil(numbram)));
      |     set_param([gcb, '/multiport_switch'],...
      |         'DataPortOrder', 'Zero-based contiguous');
      | 
      |     % Add Constant Zero
      |     add_block('hdlsllib/Sources/Constant',...
      |         [gcb, '/zero'], 'Position',...
      |         [425 -65 455 -35]);
      |     set_param([gcb, '/zero'],...
      |         'Value', int2str(0));
      |     set_param([gcb, '/zero'],...
      |         'OutDataTypeStr', ['fixdt(0, ', int2str(ceil(numbram)), ', 0)']);
      | 
      |     % Add Vector Concatenate
      |     add_block('hdlsllib/Signal Routing/Vector Concatenate',...
      |         [gcb, '/vector_concatenate'], 'Position',...
      |         [1015, -113, 1025, 38]);
      |     set_param([gcb, '/vector_concatenate'],...
      |         'NumInputs', int2str(ceil(numbram)));
      | 
      |     % Add Bitwise-OR
      |     add_block('hdlsllib/Logic and Bit Operations/Bitwise Operator',...
      |         [gcb, '/bitwise_or'], 'Position',...
      |         [1165, -54, 1205, -16]);
      |     set_param([gcb, '/bitwise_or'],...
      |         'logicop', 'OR');
      |     set_param([gcb, '/bitwise_or'],...
      |         'UseBitMask', 0);
      |     set_param([gcb, '/bitwise_or'],...
      |         'NumInputPorts', int2str(1));
      | 
      |     % Add delay for bram access
      |     add_block('hdlsllib/Discrete/Delay',...
      |         [gcb, '/delay'], 'Position',...
      |         [1248, 60, 1282, 95]);
      |     set_param([gcb, '/delay'],...
      |         'DelayLength', int2str(1));
      |     
      |     % Add bitslice
      |     add_block('hdlsllib/Logic and Bit Operations/Bit Slice',...
      |         [gcb, '/wr_bitslice'], 'Position',...
      |         [-65 180 25 220]);
      | 
      |     % Set bitslice parameters
      |     set_param([gcb, '/wr_bitslice'],...
      |         'lidx', int2str(ceil(log2(d)-1)));
      |     set_param([gcb, '/wr_bitslice'],...
      |         'ridx', int2str(log2(a(1))));
      |     
      |     % Add bitslice
      |     add_block('hdlsllib/Logic and Bit Operations/Bit Slice',...
      |         [gcb, '/rd_bitslice'], 'Position',...
      |         [-65 280 25 320]);
      | 
      |     % Set bitslice parameters
      |     set_param([gcb, '/rd_bitslice'],...
      |         'lidx', int2str(ceil(log2(d)-1)));
      |     set_param([gcb, '/rd_bitslice'],...
      |         'ridx', int2str(log2(a(1))));
      |     
      |     for i = 1:ceil(numbram)
      |         
      |         %%%%% Begin Adding Blocks %%%%%
      |         % Add Simple RAM
      |         add_block('hdlsllib/HDL RAMs/Simple Dual Port RAM',...
      |             [gcb, '/simple_ram_', int2str(i-1)], 'Position',...
      |             [635 0+600*y 635+200 400+600*y]);
      | 
      |         % Set RAM parameters
      |         set_param([gcb, '/simple_ram_', int2str(i-1)],...
      |             'ram_size', int2str(log2(a(1))));
      | 
      |         % Add compare to constant
      |         add_block('hdlsllib/Logic and Bit Operations/Compare To Constant',...
      |             [gcb, '/wr_cmp2const_', int2str(i-1)], 'Position',...
      |             [190 225+y*600 220 255+y*600]); 
      | 
      |         % Set compare to zero parameters
      |         set_param([gcb, '/wr_cmp2const_', int2str(i-1)],...
      |             'relop', '==');
      | 
      |         % Set compare to zero parameters
      |         set_param([gcb, '/wr_cmp2const_', int2str(i-1)],...
      |             'const', int2str(i-1));
      |         
      |         % Add compare to constant
      |         add_block('hdlsllib/Logic and Bit Operations/Compare To Constant',...
      |             [gcb, '/rd_cmp2const_', int2str(i-1)], 'Position',...
      |             [190 445+y*600 220 475+y*600]); 
      | 
      |         % Set compare to zero parameters
      |         set_param([gcb, '/rd_cmp2const_', int2str(i-1)],...
      |             'relop', '==');
      | 
      |         % Set compare to zero parameters
      |         set_param([gcb, '/rd_cmp2const_', int2str(i-1)],...
      |             'const', int2str(i-1));
      | 
      |         % Add and logic
      |         add_block('hdlsllib/Logic and Bit Operations/Logical Operator',...
      |             [gcb, '/and_', int2str(i-1)], 'Position',...
      |             [420 231+600*y 455 264+600*y]);
      | 
      |         % Set and logic parameters
      |         set_param([gcb, '/and_', int2str(i-1)],...
      |             'Operator', 'AND');
      | 
      |         % Add Switch
      |         add_block('hdlsllib/Signal Routing/Switch',...
      |             [gcb, '/switch_', int2str(i-1)], 'Position',...
      |             [685 -113+600*y 785 -37+600*y]);
      | 
      |         % Set switch parameters
      |         set_param([gcb, '/switch_', int2str(i-1)],...
      |             'Threshold', int2str(1));
      | 
      |         % Add Constant
      |         add_block('hdlsllib/Sources/Constant',...
      |             [gcb, '/constant_', int2str(i-1)], 'Position',...
      |             [425 -115+600*y 455 -85+600*y]);
      | 
      |         % Set Constant parameters
      |         set_param([gcb, '/constant_', int2str(i-1)],...
      |             'Value', int2str(i-1));
      |         set_param([gcb, '/constant_', int2str(i-1)],...
      |             'OutDataTypeStr', ['fixdt(0, ', int2str(ceil(numbram)), ', 0)']);   
      | 
      |         %%%%% Begin Wire Connections %%%%%        
      |         % Connect "wr_data" to "simple_ram_i"
      |         add_line(gcb, 'wr_data/1', ['simple_ram_', int2str(i-1), '/1'],...
      |             'autorouting','on');
      | 
      |         % Connect "wr_address" to "simple_ram_i"
      |         add_line(gcb, 'wr_address/1', ['simple_ram_', int2str(i-1), '/2'],...
      |             'autorouting','on');
      | 
      |         % Connect "rd_address" to "simple_ram_i"
      |         add_line(gcb, 'rd_address/1', ['simple_ram_', int2str(i-1), '/4'],...
      |             'autorouting','on');
      | 
      |         % Connect "constant_i" to "switch_i"
      |         add_line(gcb, ['constant_', int2str(i-1), '/1'], ['switch_', int2str(i-1), '/1'],...
      |             'autorouting','on');
      | 
      |         % Connect "zero" to "switch_i"
      |         add_line(gcb, 'zero/1', ['switch_', int2str(i-1), '/3'],...
      |             'autorouting','on');
      | 
      |         % Connect "switch_i" to "vector_concatenate"
      |         add_line(gcb, ['switch_', int2str(i-1), '/1'], ['vector_concatenate/', int2str(i)],...
      |             'autorouting','on');
      | 
      |         % Connect "rd_address" to "simple_ram_i"
      |         add_line(gcb, ['simple_ram_', int2str(i-1), '/1'],['multiport_switch/', int2str(i+1)],...
      |             'autorouting','on');
      | 
      |         % Connect "bitslice_i" to "wr_cmp2const_i"
      |         add_line(gcb, ['wr_bitslice/1'], ['wr_cmp2const_', int2str(i-1), '/1'],...
      |             'autorouting','on');
      |         
      |         % Connect "bitslice_i" to "rd_cmp2const_i"
      |         add_line(gcb, ['rd_bitslice/1'], ['rd_cmp2const_', int2str(i-1), '/1'],...
      |             'autorouting','on');
      | 
      |         % Connect "wr_en" to "and_i"
      |         add_line(gcb, ['wr_en/1'], ['and_', int2str(i-1), '/2'],...
      |             'autorouting','on');
      | 
      |         % Connect "and_i" to "simple_ram_0"
      |         add_line(gcb, ['and_', int2str(i-1), '/1'], ['simple_ram_', int2str(i-1), '/3'],...
      |             'autorouting','on');
      | 
      |         % Connect "wr_cmp2const_i" to "and_i"
      |         add_line(gcb, ['wr_cmp2const_', int2str(i-1), '/1'], ['and_', int2str(i-1), '/1'],...
      |             'autorouting','on');
      | 
      |         % Connect "rd_cmp2const_i" to "switch_i"
      |         add_line(gcb, ['rd_cmp2const_', int2str(i-1), '/1'], ['switch_', int2str(i-1), '/2'],...
      |             'autorouting','on');
      |          
      |         % Update coordinates
      |         y = y + 1;
      |         
      |     end
      |     
      |     % Connect "rd_addr" to "bitslice_i"
      |     add_line(gcb, ['rd_addr/1'], ['rd_bitslice/1'],...
      |         'autorouting','on');
      |     
      |     % Connect "wr_addr" to "bitslice_i"
      |     add_line(gcb, ['wr_addr/1'], ['wr_bitslice/1'],...
      |         'autorouting','on');
      |     
      |     % Connect "wr_addr" to "wr_address"
      |     add_line(gcb, 'wr_addr/1', ['wr_address', '/1'],...
      |         'autorouting','on');
      | 
      |     % Connect "rd_addr" to "rd_address"
      |     add_line(gcb, 'rd_addr/1', ['rd_address', '/1'],...
      |         'autorouting','on');
      | 
      |     % Connect "vector_concatenate" to "bitwise_or"
      |     add_line(gcb, ['vector_concatenate/1'], ['bitwise_or/1'],...
      |         'autorouting','on');
      | 
      |     % Connect "bitwise_or" to "delay"
      |     add_line(gcb, ['bitwise_or/1'], ['delay/1'],...
      |         'autorouting','on');
      | 
      |     % Connect "delay" to "multiport_switch"
      |     add_line(gcb, ['delay/1'], ['multiport_switch/1'],...
      |         'autorouting','on');
      | 
      |     % Connect "multiport_switch" to "rd_data"
      |     add_line(gcb, ['multiport_switch/1'], ['rd_data/1'],...
      |         'autorouting','on');
      |     
      | end
      | 
      | % If there is a half bram we must change a few parameters. Firstly, delete
      | % the write and read address lines. Then add bitslice blocks to reduce the
      | % address space in half. Connect rd_addr and wr_addr to the corresponding ports
      | % on the bram. Finally, change the address depth.
      | if halfbram
      |     
      |     if ceil(numbram) > 1
      |         
      |         % Delete lines
      |         delete_line(gcb, ['wr_address/1'], ['simple_ram_', int2str(i-1), '/2'])
      |         delete_line(gcb, ['rd_address/1'], ['simple_ram_', int2str(i-1), '/4'])
      |         
      |         % Write Address half ram Slice
      |         add_block('hdlsllib/Logic and Bit Operations/Bit Slice',...
      |                 [gcb, '/wr_address_hr'], 'Position',...
      |                 [160 130+(y-1)*600 250 170+(y-1)*600]);
      |         % Set bitslice parameters
      |         set_param([gcb, '/wr_address_hr'],...
      |             'lidx', int2str(log2(a(1))-2));
      |         set_param([gcb, '/wr_address_hr'],...
      |             'ridx', int2str(0));
      | 
      |         % Read Address half ram Slice
      |         add_block('hdlsllib/Logic and Bit Operations/Bit Slice',...
      |                 [gcb, '/rd_address_hr'], 'Position',...
      |                 [160 330+(y-1)*600 250 370+(y-1)*600]);
      |         % Set bitslice parameters
      |         set_param([gcb, '/rd_address_hr'],...
      |             'lidx', int2str(log2(a(1))-2));
      |         set_param([gcb, '/rd_address_hr'],...
      |             'ridx', int2str(0));
      | 
      |         % Connect "wr_addr" to "wr_address_hr"
      |         add_line(gcb, 'wr_addr/1', ['wr_address_hr', '/1'],...
      |             'autorouting','on');
      | 
      |         % Connect "rd_addr" to "rd_address_hr"
      |         add_line(gcb, 'rd_addr/1', ['rd_address_hr', '/1'],...
      |             'autorouting','on');
      | 
      |         % Connect "wr_address_hr" to "simple_ram_i"
      |         add_line(gcb, ['wr_address_hr', '/1'], ['simple_ram_', int2str(i-1), '/2'],...
      |             'autorouting','on');
      | 
      |         % Connect "rd_address_hr" to "simple_ram_i"
      |         add_line(gcb, ['rd_address_hr', '/1'], ['simple_ram_', int2str(i-1), '/4'],...
      |             'autorouting','on');
      | 
      |     else
      |         % Set bitslice parameters
      |         set_param([gcb, '/wr_address'],...
      |             'lidx', int2str(log2(a(1))-2));
      |         set_param([gcb, '/wr_address'],...
      |             'ridx', int2str(0));
      |         % Set bitslice parameters
      |         set_param([gcb, '/rd_address'],...
      |             'lidx', int2str(log2(a(1))-2));
      |         set_param([gcb, '/rd_address'],...
      |             'ridx', int2str(0));
      |         
      |     end
      |     
      |     % Update the ram parameters (address bits)
      |     set_param([gcb, '/simple_ram_', int2str(i-1)],...
      |         'ram_size', int2str(log2(a(1)/2)));
      |     
      | end
      | 
      | b_hidden = b;
      | d_hiddne = d;
  rd_data : Outport

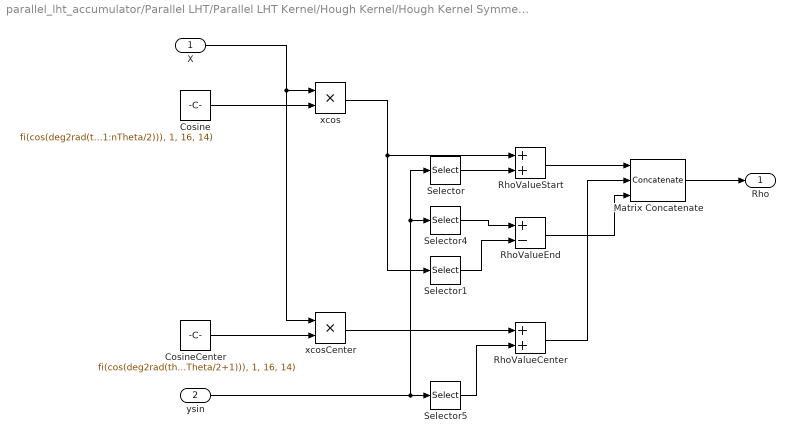
== system parallel_lht_accumulator/Parallel LHT/Parallel LHT Kernel/Hough Kernel/Hough Kernel Symmetric Look Ahead/Hough Kernel Symmetric ==
  X : Inport
  ysin : Inport  Port=2
  Cosine : Constant  Value=fi(cos(deg2rad(theta(1:nTheta/2))), 1, 16, 14)  VectorParams1D=off  OutDataTypeStr=fixdt(1,16,14)  SampleTime=-1
  CosineCenter : Constant  Value=fi(cos(deg2rad(theta(nTheta/2+1))), 1, 16, 14)  VectorParams1D=off  OutDataTypeStr=fixdt(1,16,14)  SampleTime=-1
  Matrix Concatenate : Concatenate  NumInputs=3  Mode=Multidimensional array  ConcatenateDimension=2
  RhoValueCenter : Sum  OutDataTypeStr=fixdt(1, ceil(log2(2*maxRho)), 0);  RndMeth=Round
  RhoValueEnd : Sum  Inputs=+-  OutDataTypeStr=fixdt(1, ceil(log2(2*maxRho)), 0);  RndMeth=Round
  RhoValueStart : Sum  OutDataTypeStr=fixdt(1, ceil(log2(2*maxRho)), 0);  RndMeth=Round
  Selector : Selector  NumberOfDimensions=2  IndexMode=Zero-based  InputPortWidth=3  IndexOptions=Index vector (dialog),Index vector (dialog)  Indices=0,[0:1:nTheta/2-1]  OutputSizes=1,1
  Selector1 : Selector  NumberOfDimensions=2  IndexMode=Zero-based  InputPortWidth=3  IndexOptions=Index vector (dialog),Index vector (dialog)  Indices=0,uint32([nTheta/2-1:-1:1])  OutputSizes=1,1
  Selector4 : Selector  NumberOfDimensions=2  IndexMode=Zero-based  InputPortWidth=3  IndexOptions=Index vector (dialog),Index vector (dialog)  Indices=0,uint32([nTheta/2-1:-1:1])  OutputSizes=1,1
  Selector5 : Selector  NumberOfDimensions=2  IndexMode=Zero-based  InputPortWidth=3  IndexOptions=Index vector (dialog),Index vector (dialog)  Indices=0,uint32([nTheta/2])  OutputSizes=1,1
  xcos : Product  OutDataTypeStr=fixdt(1, ceil(log2(width)), 0);  RndMeth=Round
  xcosCenter : Product  OutDataTypeStr=fixdt(1, ceil(log2(width)), 0);  RndMeth=Round
  Rho : Outport  VectorParamsAs1DForOutWhenUnconnected=off
  wires:
  Selector/1 -> RhoValueStart/2
  Selector5/1 -> RhoValueCenter/2
  ysin/1 -> Selector5/1, Selector/1, Selector4/1
  Selector4/1 -> RhoValueEnd/1
  xcosCenter/1 -> RhoValueCenter/1
  CosineCenter/1 -> xcosCenter/2
  Cosine/1 -> xcos/2
  X/1 -> xcos/1, xcosCenter/1
  xcos/1 -> RhoValueStart/1, Selector1/1
  RhoValueEnd/1 -> Matrix Concatenate/3
  RhoValueStart/1 -> Matrix Concatenate/1
  Matrix Concatenate/1 -> Rho/1
  RhoValueCenter/1 -> Matrix Concatenate/2
  Selector1/1 -> RhoValueEnd/2
